simulink model "model_translational_wind"  (R2020b)
settings: Solver=VariableStepAuto  StartTime=0.0  StopTime=10.0  RelTol=1e-3
undefined symbols (not defined in the file or in its folder): trans_height_end, trans_height_start, trans_lat_end, trans_lat_start, trans_lon_end, trans_lon_start, translationalWind
settings Model: Creator=C:\Users\Dogukan  LastModifiedBy=C:\Users\Dogukan

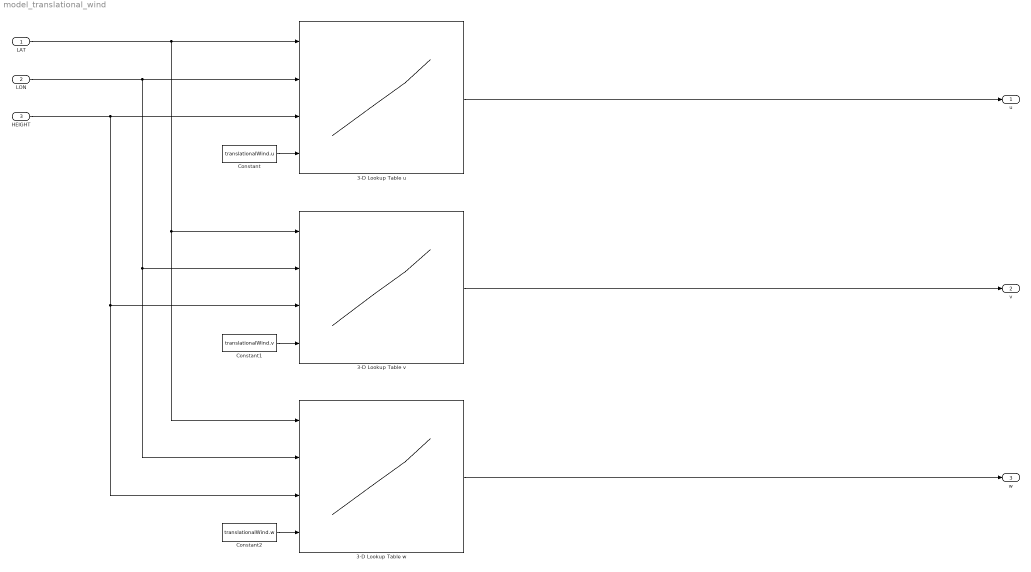
== system model_translational_wind ==
  LAT : Inport
  LON : Inport  Port=2
  HEIGHT : Inport  Port=3
  3-D Lookup Table u : Lookup_n-D  NumberOfTableDimensions=3  BreakpointsForDimension1=[trans_lat_start, trans_lat_start+1E-08, trans_lat_end-1E-08, trans_lat_end]  BreakpointsForDimension2=[trans_lon_start, trans_lon_start+1E-08, trans_lon_end-1E-08, trans_lon_end]  BreakpointsForDimension3=[trans_height_start, trans_height_start+1E-08, trans_height_end-1E-08, trans_height_end]  TableSource=Input port  Table=reshape(repmat([4 5 6;16 19 20;10 18 23],1,2),[3,3,2])  ExtrapMethod=Clip  InternalRulePriority=Speed  RndMeth=Simplest  InputSameDT=on
      settings: InputPortMap=u0,u1,u2,p221
  3-D Lookup Table v : Lookup_n-D  NumberOfTableDimensions=3  BreakpointsForDimension1=[trans_lat_start, trans_lat_start+1E-08, trans_lat_end-1E-08, trans_lat_end]  BreakpointsForDimension2=[trans_lon_start, trans_lon_start+1E-08, trans_lon_end-1E-08, trans_lon_end]  BreakpointsForDimension3=[trans_height_start, trans_height_start+1E-08, trans_height_end-1E-08, trans_height_end]  TableSource=Input port  Table=reshape(repmat([4 5 6;16 19 20;10 18 23],1,2),[3,3,2])  ExtrapMethod=Clip  InternalRulePriority=Speed  RndMeth=Simplest  InputSameDT=on
      settings: InputPortMap=u0,u1,u2,p221
  3-D Lookup Table w : Lookup_n-D  NumberOfTableDimensions=3  BreakpointsForDimension1=[trans_lat_start, trans_lat_start+1E-08, trans_lat_end-1E-08, trans_lat_end]  BreakpointsForDimension2=[trans_lon_start, trans_lon_start+1E-08, trans_lon_end-1E-08, trans_lon_end]  BreakpointsForDimension3=[trans_height_start, trans_height_start+1E-08, trans_height_end-1E-08, trans_height_end]  TableSource=Input port  Table=reshape(repmat([4 5 6;16 19 20;10 18 23],1,2),[3,3,2])  ExtrapMethod=Clip  InternalRulePriority=Speed  RndMeth=Simplest  InputSameDT=on
      settings: InputPortMap=u0,u1,u2,p221
  Constant : Constant  Value=translationalWind.u
  Constant1 : Constant  Value=translationalWind.v
  Constant2 : Constant  Value=translationalWind.w
  u : Outport
  v : Outport  Port=2
  w : Outport  Port=3
  wires:
  Constant/1 -> 3-D Lookup Table u/4
  Constant1/1 -> 3-D Lookup Table v/4
  Constant2/1 -> 3-D Lookup Table w/4
  LAT/1 -> 3-D Lookup Table w/1, 3-D Lookup Table v/1, 3-D Lookup Table u/1
  LON/1 -> 3-D Lookup Table w/2, 3-D Lookup Table v/2, 3-D Lookup Table u/2
  HEIGHT/1 -> 3-D Lookup Table w/3, 3-D Lookup Table v/3, 3-D Lookup Table u/3
  3-D Lookup Table u/1 -> u/1
  3-D Lookup Table v/1 -> v/1
  3-D Lookup Table w/1 -> w/1
